simulink model "Speed_LegacyComparison"  (R2022a)
settings: Solver=VariableStepAuto  StartTime=0.0  StopTime=10.0  RelTol=1e-3
undefined symbols (not defined in the file or in its folder): d, F_0, F_0k, g, m, M, P_0, P_0k, PD_s, PI, PI_s, Ts, V_0, V_0k
settings Model: Creator=DELL  LastModifiedBy=DELL

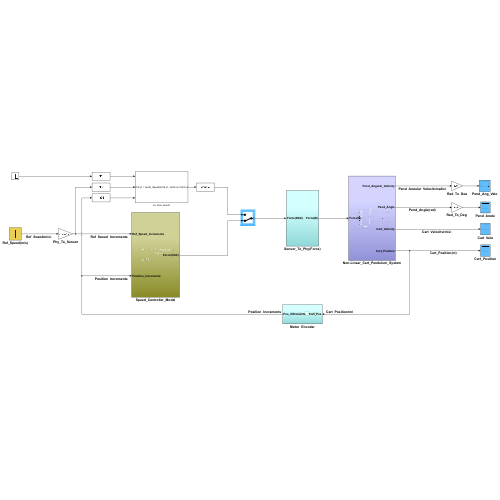
[thumbnail: Simulink's stored preview of the top-level diagram]
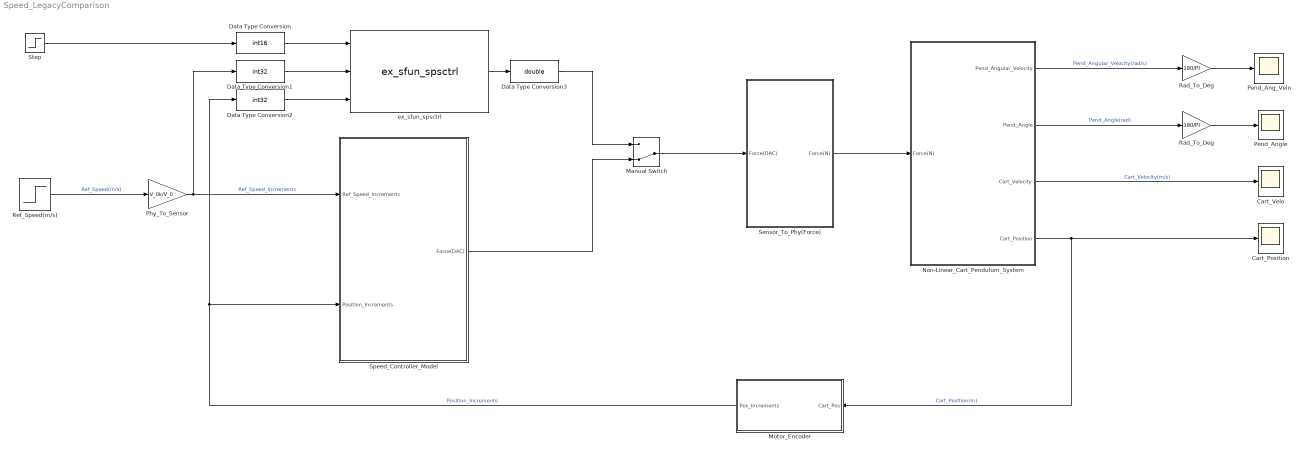
== system Speed_LegacyComparison ==
  Cart_Position : Scope
  Cart_Velo : Scope
  Data Type Conversion : DataTypeConversion  OutDataTypeStr=int16  SaturateOnIntegerOverflow=off  RndMeth=Floor
  Data Type Conversion1 : DataTypeConversion  OutDataTypeStr=int32  SaturateOnIntegerOverflow=off  RndMeth=Floor
  Data Type Conversion2 : DataTypeConversion  OutDataTypeStr=int32  SaturateOnIntegerOverflow=off  RndMeth=Floor
  Data Type Conversion3 : DataTypeConversion  OutDataTypeStr=double  SaturateOnIntegerOverflow=off  RndMeth=Floor
  Manual Switch : ManualSwitch  CurrentSetting=0
  Motor_Encoder : Subsystem
  Non-Linear_Cart_Pendulum_System : Subsystem
  Pend_Ang_Velo : Scope
  Pend_Angle : Scope
  Phy_To_Sensor : Gain  Gain=V_0k/V_0
  Rad_To_Deg : Gain  Gain=180/PI
  "Rad_To_Deg " : Gain  Gain=180/PI
  Ref_Speed(m/s) : Step  After=0.5  SampleTime=Ts
  Sensor_To_Phy(Force) : Subsystem
  Speed_Controller_Model : Subsystem
  Step : Step  Time=2*Ts  Before=1  After=0  SampleTime=Ts
  ex_sfun_spsctrl : S-Function  FunctionName=ex_sfun_spsctrl  SFunctionDeploymentMode=off  EnableBusSupport=off  mask(Legacy Function){SFunctionSpec=int16 y1 = spctrl_Speed(int16 u1, int32 u2, int32 u3), ShowSpec=on}
      mask prompts: ShowSpec "Display function specification"
      mask help:
      | This block allows you to call the legacy functions specified by the following Legacy Code Tool definition:
      | def.SFunctionName = 'ex_sfun_spsctrl';
      | def.OutputFcnSpec = 'int16 y1 = spctrl_Speed(int16 u1, int32 u2, int32 u3)';
      | def.HeaderFiles = {'xil_types.h', 'Fixedpt_Speed_Control.h'};
      mask Help: <p>This block was generated automatically by the Legacy Code Tool. For detailed help on this tool, call<a href="matlab:legacy_code('help')"> legacy_code('help')</a>.</p>
      mask Callback ShowSpec:
      | if strcmp(get_param(gcbh, 'ShowSpec'), 'on')
      |   set_param(gcbh, 'MaskDisplay', sprintf('fprintf(''%s'');', get_param(gcbh, 'SFunctionSpec')));
      | else
      |   set_param(gcbh, 'MaskDisplay', sprintf('fprintf(''%s'');', get_param(gcbh, 'FunctionName')));
      | end
      mask Display: fprintf('int16 y1 = spctrl_Speed(int16 u1, int32 u2, int32 u3)');
  wires:
  Non-Linear_Cart_Pendulum_System/4(Cart_Position) -> Motor_Encoder/1(Cart_Pos), Cart_Position/1  "Cart_Position(m)"
  Phy_To_Sensor/1 -> Data Type Conversion1/1, Speed_Controller_Model/1(Ref_Speed_Increments)  "Ref_Speed_Increments"
  Non-Linear_Cart_Pendulum_System/2(Pend_Angle) -> "Rad_To_Deg "/1  "Pend_Angle(rad)"
  Non-Linear_Cart_Pendulum_System/3(Cart_Velocity) -> Cart_Velo/1  "Cart_Velocity(m/s)"
  Sensor_To_Phy(Force)/1(Force(N)) -> Non-Linear_Cart_Pendulum_System/1(Force(N))
  "Rad_To_Deg "/1 -> Pend_Angle/1
  Rad_To_Deg/1 -> Pend_Ang_Velo/1
  Motor_Encoder/1(Pos_Increments) -> Data Type Conversion2/1, Speed_Controller_Model/2(Position_Increments)  "Position_Increments"
  Non-Linear_Cart_Pendulum_System/1(Pend_Angular_Velocity) -> Rad_To_Deg/1  "Pend_Angular_Velocity(rad/s)"
  Ref_Speed(m/s)/1 -> Phy_To_Sensor/1  "Ref_Speed(m/s)"
  Data Type Conversion/1 -> ex_sfun_spsctrl/1
  Data Type Conversion1/1 -> ex_sfun_spsctrl/2
  Data Type Conversion2/1 -> ex_sfun_spsctrl/3
  Step/1 -> Data Type Conversion/1
  ex_sfun_spsctrl/1 -> Data Type Conversion3/1
  Data Type Conversion3/1 -> Manual Switch/1
  Speed_Controller_Model/1(Force(DAC)) -> Manual Switch/2
  Manual Switch/1 -> Sensor_To_Phy(Force)/1(Force(DAC))

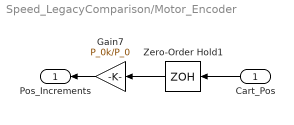
== system Speed_LegacyComparison/Motor_Encoder ==
  Cart_Pos : Inport
  Gain7 : Gain  Gain=P_0k/P_0
  Zero-Order Hold1 : ZeroOrderHold  SampleTime=Ts
  Pos_Increments : Outport
  wires:
  Gain7/1 -> Pos_Increments/1
  Zero-Order Hold1/1 -> Gain7/1
  Cart_Pos/1 -> Zero-Order Hold1/1

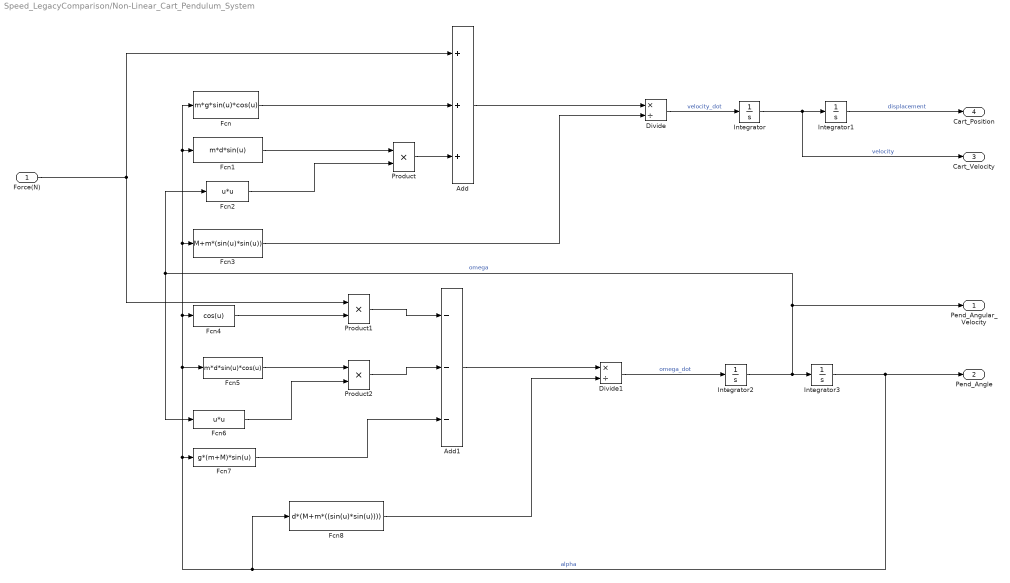
== system Speed_LegacyComparison/Non-Linear_Cart_Pendulum_System ==
  Force(N) : Inport
  Add : Sum  Inputs=+++
  Add1 : Sum  Inputs=---
  Divide : Product  Inputs=*/
  Divide1 : Product  Inputs=*/
  Fcn : Fcn  Expr=m*g*sin(u)*cos(u)
  Fcn1 : Fcn  Expr=m*d*sin(u)
  Fcn2 : Fcn  Expr=u*u
  Fcn3 : Fcn  Expr=M+m*(sin(u)*sin(u))
  Fcn4 : Fcn  Expr=cos(u)
  Fcn5 : Fcn  Expr=m*d*sin(u)*cos(u)
  Fcn6 : Fcn  Expr=u*u
  Fcn7 : Fcn  Expr=g*(m+M)*sin(u)
  Fcn8 : Fcn  Expr=d*(M+m*((sin(u)*sin(u))))
  Integrator{,1..3} (4 alike) : Integrator
  Product : Product
  Product1 : Product
  Product2 : Product
  Pend_Angular_Velocity : Outport  VectorParamsAs1DForOutWhenUnconnected=off
  Pend_Angle : Outport  Port=2  VectorParamsAs1DForOutWhenUnconnected=off
  Cart_Velocity : Outport  Port=3  VectorParamsAs1DForOutWhenUnconnected=off
  Cart_Position : Outport  Port=4  VectorParamsAs1DForOutWhenUnconnected=off
  wires:
  Add/1 -> Divide/1
  Integrator2/1 -> Integrator3/1, Pend_Angular_Velocity/1, Fcn2/1, Fcn6/1  "omega"
  Fcn1/1 -> Product/1
  Integrator1/1 -> Cart_Position/1  "displacement"
  Fcn6/1 -> Product2/2
  Product/1 -> Add/3
  Fcn2/1 -> Product/2
  Fcn4/1 -> Product1/2
  Fcn/1 -> Add/2
  Integrator3/1 -> Pend_Angle/1, Fcn8/1, Fcn7/1, Fcn5/1, Fcn4/1, Fcn/1, Fcn1/1, Fcn3/1  "alpha"
  Divide/1 -> Integrator/1  "velocity_dot"
  Fcn3/1 -> Divide/2
  Product2/1 -> Add1/2
  Add1/1 -> Divide1/1
  Fcn5/1 -> Product2/1
  Product1/1 -> Add1/1
  Fcn8/1 -> Divide1/2
  Fcn7/1 -> Add1/3
  Force(N)/1 -> Add/1, Product1/1
  Integrator/1 -> Integrator1/1, Cart_Velocity/1  "velocity"
  Divide1/1 -> Integrator2/1  "omega_dot"

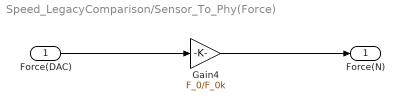
== system Speed_LegacyComparison/Sensor_To_Phy(Force) ==
  Force(DAC) : Inport
  Gain4 : Gain  Gain=F_0/F_0k
  Force(N) : Outport
  wires:
  Force(DAC)/1 -> Gain4/1
  Gain4/1 -> Force(N)/1

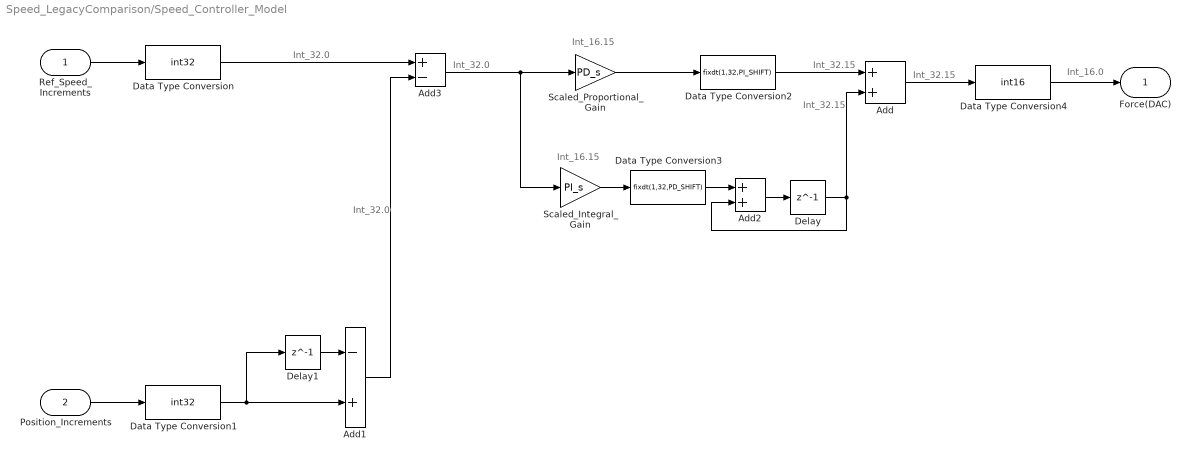
== system Speed_LegacyComparison/Speed_Controller_Model ==
  note: Int_32.0
  note: Int_32.0
  note: Int_32.0
  note: Int_32.15
  note: Int_32.15
  note: Int_32.15
  note: Int_16.0
  note: Int_16.15
  note: Int_16.15
  Ref_Speed_Increments : Inport
  Position_Increments : Inport  Port=2
  Add : Sum
  Add1 : Sum  Inputs=-+
  Add2 : Sum
  Add3 : Sum  Inputs=+-
  Data Type Conversion : DataTypeConversion  OutDataTypeStr=int32  SaturateOnIntegerOverflow=off  RndMeth=Floor
  Data Type Conversion1 : DataTypeConversion  OutDataTypeStr=int32  SaturateOnIntegerOverflow=off  RndMeth=Floor
  Data Type Conversion2 : DataTypeConversion  OutDataTypeStr=fixdt(1,32,PI_SHIFT)  SaturateOnIntegerOverflow=off  RndMeth=Floor
  Data Type Conversion3 : DataTypeConversion  OutDataTypeStr=fixdt(1,32,PD_SHIFT)  SaturateOnIntegerOverflow=off  RndMeth=Floor
  Data Type Conversion4 : DataTypeConversion  OutDataTypeStr=int16  SaturateOnIntegerOverflow=off  RndMeth=Floor
  Delay : Delay  DelayLength=1  SampleTime=Ts
  Delay1 : Delay  DelayLength=1  SampleTime=Ts
  Scaled_Integral_Gain : Gain  Gain=PI_s
  Scaled_Proportional_Gain : Gain  Gain=PD_s
  Force(DAC) : Outport
  wires:
  Add2/1 -> Delay/1
  Scaled_Integral_Gain/1 -> Data Type Conversion3/1
  Scaled_Proportional_Gain/1 -> Data Type Conversion2/1
  Delay/1 -> Add/2, Add2/2
  Add3/1 -> Scaled_Integral_Gain/1, Scaled_Proportional_Gain/1
  Add/1 -> Data Type Conversion4/1
  Ref_Speed_Increments/1 -> Data Type Conversion/1
  Add1/1 -> Add3/2
  Delay1/1 -> Add1/1
  Position_Increments/1 -> Data Type Conversion1/1
  Data Type Conversion/1 -> Add3/1
  Data Type Conversion1/1 -> Delay1/1, Add1/2
  Data Type Conversion2/1 -> Add/1
  Data Type Conversion3/1 -> Add2/1
  Data Type Conversion4/1 -> Force(DAC)/1
